simulink model "yori_coba_variabel_m_file"  (R2023a)
settings: Solver=VariableStepAuto  StartTime=0.0  StopTime=10.0  RelTol=1e-3
values from neighbouring files (symbols this model uses):
  dxdt_init = 0    [matlab.mat]
  k = 2    [matlab.mat]
  m = 20    [matlab.mat]
  x_init = 4    [matlab.mat]
settings Model: Creator=HP  LastModifiedBy=HP

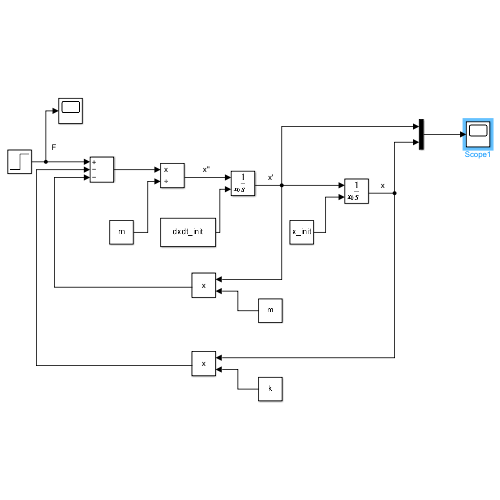
[thumbnail: Simulink's stored preview of the top-level diagram]
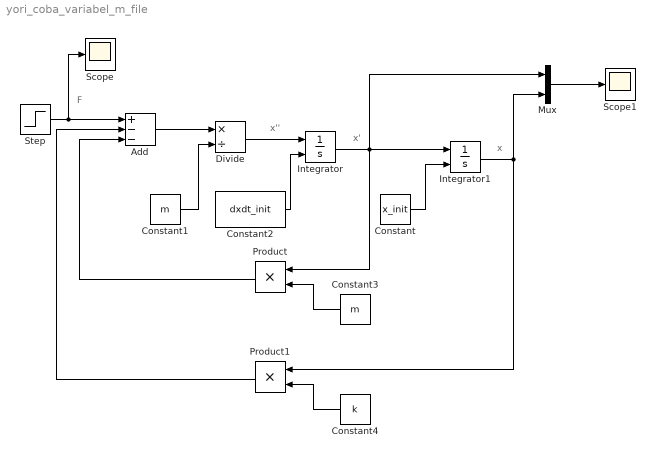
== system yori_coba_variabel_m_file ==
  note: F
  note: x
  note: x'
  note: x''
  Add : Sum  Inputs=+--
  Constant : Constant  Value=x_init
  Constant1 : Constant  Value=m
  Constant2 : Constant  Value=dxdt_init
  Constant3 : Constant  Value=m
  Constant4 : Constant  Value=k
  Divide : Product  Inputs=*/
  Integrator : Integrator  InitialConditionSource=external
  Integrator1 : Integrator  InitialConditionSource=external
  Mux : Mux  Inputs=2
  Product : Product
  Product1 : Product
  Scope : Scope
  Scope1 : Scope
  Step : Step  SampleTime=0
  wires:
  Step/1 -> Add/1, Scope/1
  Add/1 -> Divide/1
  Constant1/1 -> Divide/2
  Divide/1 -> Integrator/1
  Constant2/1 -> Integrator/2
  Integrator/1 -> Product/1, Integrator1/1, Mux/1
  Constant/1 -> Integrator1/2
  Mux/1 -> Scope1/1
  Integrator1/1 -> Mux/2, Product1/1
  Constant3/1 -> Product/2
  Constant4/1 -> Product1/2
  Product1/1 -> Add/2
  Product/1 -> Add/3
